simulink library "SimWindFarm_lib"  (Simulink 10.3)
settings: Solver=ode45  StartTime=0.0  StopTime=10.0  RelTol=1e-3  EnableMultiTasking=on
undefined symbols (not defined in the file): sigbuilder_block
libraries: simulink x3
(part 2 of 2)

== system SimWindFarm_lib/Farm Template - No Taylor Added Turbulence/Post processing ==
  Fatigue Computation : Subsystem
      settings: OpenFcn=fatigue=fatiguegui(logsout);
      mask Display: image(imread('rainflow.png'))

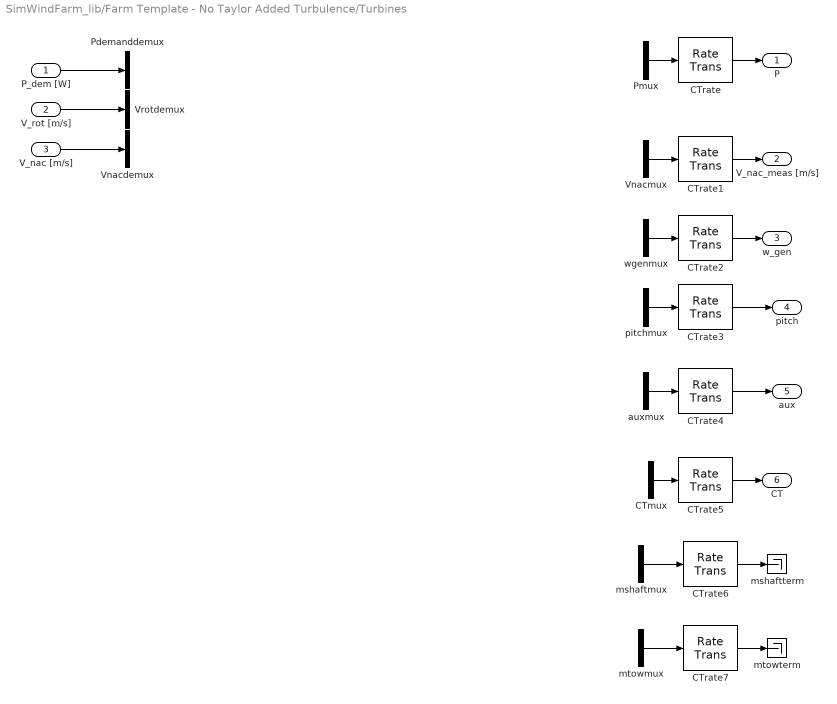
== system SimWindFarm_lib/Farm Template - No Taylor Added Turbulence/Turbines ==
  P_dem [W] : Inport
  V_rot [m/s] : Inport  Port=2
  V_nac [m/s] : Inport  Port=3
  CTmux : Mux  Inputs=2
  CTrate{,1..7} (8 alike) : RateTransition  Deterministic=off  OutPortSampleTime=TTs
  Pdemanddemux : Demux  Outputs=3
  Pmux : Mux  Inputs=2
  Vnacdemux : Demux  Outputs=3
  Vnacmux : Mux  Inputs=2
  Vrotdemux : Demux  Outputs=3
  auxmux : Mux  Inputs=2
  mshaftmux : Mux  Inputs=2
  mshaftterm : Terminator
  mtowmux : Mux  Inputs=2
  mtowterm : Terminator
  pitchmux : Mux  Inputs=2
  wgenmux : Mux  Inputs=2
  P : Outport
  V_nac_meas [m/s] : Outport  Port=2
  w_gen : Outport  Port=3
  pitch : Outport  Port=4
  aux : Outport  Port=5
  CT : Outport  Port=6
  wires:
  V_nac [m/s]/1 -> Vnacdemux/1
  P_dem [W]/1 -> Pdemanddemux/1
  V_rot [m/s]/1 -> Vrotdemux/1
  Pmux/1 -> CTrate/1
  CTmux/1 -> CTrate5/1
  Vnacmux/1 -> CTrate1/1
  pitchmux/1 -> CTrate3/1
  auxmux/1 -> CTrate4/1
  wgenmux/1 -> CTrate2/1
  mshaftmux/1 -> CTrate6/1
  mtowmux/1 -> CTrate7/1
  CTrate/1 -> P/1
  CTrate1/1 -> V_nac_meas [m/s]/1
  CTrate2/1 -> w_gen/1
  CTrate3/1 -> pitch/1
  CTrate4/1 -> aux/1
  CTrate5/1 -> CT/1
  CTrate6/1 -> mshaftterm/1
  CTrate7/1 -> mtowterm/1

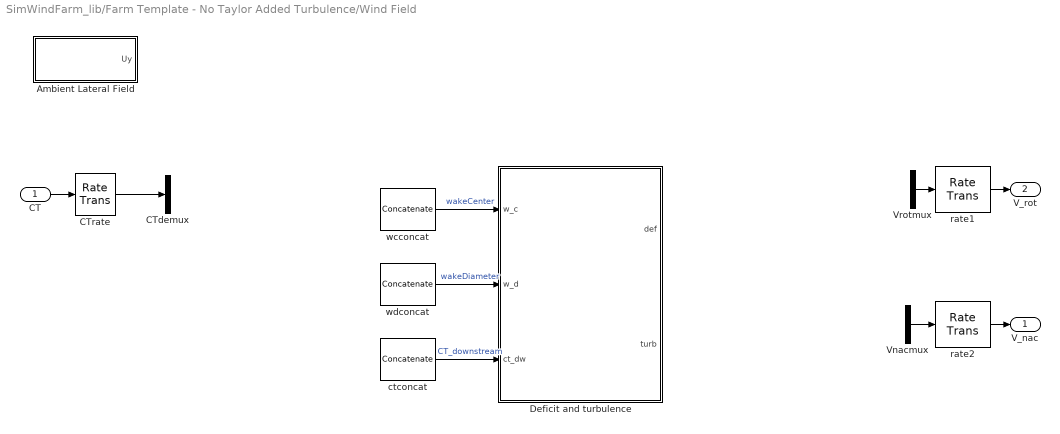
== system SimWindFarm_lib/Farm Template - No Taylor Added Turbulence/Wind Field ==
  CT : Inport
  Ambient Lateral Field : Subsystem
      mask init:
      | wind=get_param(gcb,'UserData');
  CTdemux : Demux  Outputs=3
  CTrate : RateTransition  Deterministic=off  OutPortSampleTime=10
  Deficit and turbulence : MATLAB Function  TreatAsAtomicUnit=on
  Vnacmux : Mux  Inputs=2
  Vrotmux : Mux  Inputs=2
  ctconcat : Concatenate  Mode=Multidimensional array  ConcatenateDimension=2
  rate1 : RateTransition  Deterministic=off  OutPortSampleTime=SWFTTs
  rate2 : RateTransition  Deterministic=off  OutPortSampleTime=SWFTTs
  wcconcat : Concatenate  Mode=Multidimensional array  ConcatenateDimension=2
  wdconcat : Concatenate  Mode=Multidimensional array  ConcatenateDimension=2
  V_nac : Outport
  V_rot : Outport  Port=2
  wires:
  rate2/1 -> V_nac/1
  rate1/1 -> V_rot/1
  Vnacmux/1 -> rate2/1
  Vrotmux/1 -> rate1/1
  ctconcat/1 -> Deficit and turbulence/3(ct_dw)  "CT_downstream"
  wdconcat/1 -> Deficit and turbulence/2(w_d)  "wakeDiameter"
  wcconcat/1 -> Deficit and turbulence/1(w_c)  "wakeCenter"
  CT/1 -> CTrate/1
  CTrate/1 -> CTdemux/1

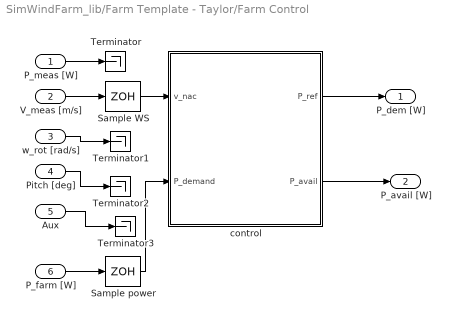
== system SimWindFarm_lib/Farm Template - Taylor/Farm Control ==
  P_meas [W] : Inport
  V_meas [m/s] : Inport  Port=2
  w_rot [rad/s] : Inport  Port=3
  Pitch [deg] : Inport  Port=4
  " Aux" : Inport  Port=5
  P_farm [W] : Inport  Port=6
  Sample WS : ZeroOrderHold  SampleTime=CTs
  Sample power : ZeroOrderHold  SampleTime=CTs
  Terminator{,1..3} (4 alike) : Terminator
  control : MATLAB Function  TreatAsAtomicUnit=on
  P_dem [W] : Outport
  P_avail [W] : Outport  Port=2
  wires:
  P_farm [W]/1 -> Sample power/1
  control/1(P_ref) -> P_dem [W]/1
  control/2(P_avail) -> P_avail [W]/1
  Sample power/1 -> control/2(P_demand)
  V_meas [m/s]/1 -> Sample WS/1
  Sample WS/1 -> control/1(v_nac)
  P_meas [W]/1 -> Terminator/1
  w_rot [rad/s]/1 -> Terminator1/1
  Pitch [deg]/1 -> Terminator2/1
  " Aux"/1 -> Terminator3/1

== system SimWindFarm_lib/Farm Template - Taylor/Grid ==
  Generated Power [W] : Inport
  Consumed Power [W] : Inport  Port=2
  Active power diff to freq : Gain  Gain=frequencygain
  Integrator : Integrator  InitialCondition=50  LimitOutput=on  UpperSaturationLimit=100  LowerSaturationLimit=0
  Sum1 : Sum  Inputs=|+-
  Grid Frequency [Hz] : Outport
  wires:
  Integrator/1 -> Grid Frequency [Hz]/1
  Sum1/1 -> Active power diff to freq/1
  Active power diff to freq/1 -> Integrator/1
  Generated Power [W]/1 -> Sum1/1
  Consumed Power [W]/1 -> Sum1/2

== system SimWindFarm_lib/Farm Template - Taylor/Network Load ==
  Power Load : Subsystem  Tag=STV Subsys  LoadFcn=sigbuilder_block('load');  StartFcn=sigbuilder_block('start');  StopFcn=sigbuilder_block('stop');  ClipboardFcn=sigbuilder_block('clipboard');  mask(Sigbuilder block){tuvar=[0:10]}
      mask help: Sigbuilder GUI
      mask init:
      | if ~strcmp(get_param(bdroot(gcbh),'SimulationStatus'),'stopped') tuvar = sigbuilder_block('maskInit'); end
      settings: CopyFcn=sigbuilder_block('copy');  DeleteFcn=sigbuilder_block('delete');  ModelCloseFcn=sigbuilder_block('modelClose');  PreSaveFcn=sigbuilder_block('preSave');  PauseFcn=sigbuilder_block('pause')  ContinueFcn=sigbuilder_block('continue')  NameChangeFcn=sigbuilder_block('namechange');  OpenFcn=sigbuilder_block('open',[437.6 199.2 550.4 400 ]);  CloseFcn=sigbuilder_block('close');
      mask Display: plot(0, 0, 100, 100,[2, 2, 32, 32, 2], [68, 8, 8, 68, 68],[32, 2], [38, 38], [32, 19, 2],[53, 60, 44], [32, 17, 17, 2],[16, 16, 31, 31]);txt = getActiveGroup(gcbh);text(2, 100, txt,'verticalAlignment', 'top');
  To rated farm power : Gain  Gain=maxpower
  Power Consumption [W] : Outport
  wires:
  Power Load/1(Signal 1) -> To rated farm power/1
  To rated farm power/1 -> Power Consumption [W]/1

== system SimWindFarm_lib/Farm Template - Taylor/Network Operator ==
  P_avail [W] : Inport
  Freq [Hz] : Inport  Port=2
  F_meas delay : TransportDelay  DelayTime=parm.delay
  Network Operator : MATLAB Function  TreatAsAtomicUnit=on
  P meas delay : TransportDelay  DelayTime=parm.delay
  Reference delay : TransportDelay  DelayTime=.01
  Sample frequency : ZeroOrderHold  SampleTime=parm.Ts
  Sample power : ZeroOrderHold  SampleTime=parm.Ts
  Unit Delay : UnitDelay  SampleTime=parm.Ts  HasFrameUpgradeWarning=on
  settings : Constant  Value=parm.settings  OutDataTypeStr=double  SampleTime=parm.Ts
  P_farm [W] : Outport
  wires:
  Freq [Hz]/1 -> Sample frequency/1
  Unit Delay/1 -> Network Operator/4(P_demand0)
  Sample frequency/1 -> F_meas delay/1  "f"
  settings/1 -> Network Operator/2(settings)  "settings"
  Sample power/1 -> P meas delay/1
  P_avail [W]/1 -> Sample power/1
  Network Operator/1(P_demand) -> Unit Delay/1, Reference delay/1
  F_meas delay/1 -> Network Operator/3(f)
  P meas delay/1 -> Network Operator/1(P_avail)
  Reference delay/1 -> P_farm [W]/1

== system SimWindFarm_lib/Farm Template - Taylor/Post processing ==
  Fatigue Computation : Subsystem
      settings: OpenFcn=fatigue=fatiguegui(logsout);
      mask Display: image(imread('rainflow.png'))
  Wake Animation : Subsystem
      settings: OpenFcn=|
      | sys=bdroot(gcb);
      | create_wakeanim(sys,logsout);
      mask Display: image(imread('wakeanim.png'))
  Wind Field Animation : Subsystem
      settings: OpenFcn=|
      | sys=bdroot(gcb);
      | windanim(sys,logsout);
      mask Display: image(imread('windanim.png'))

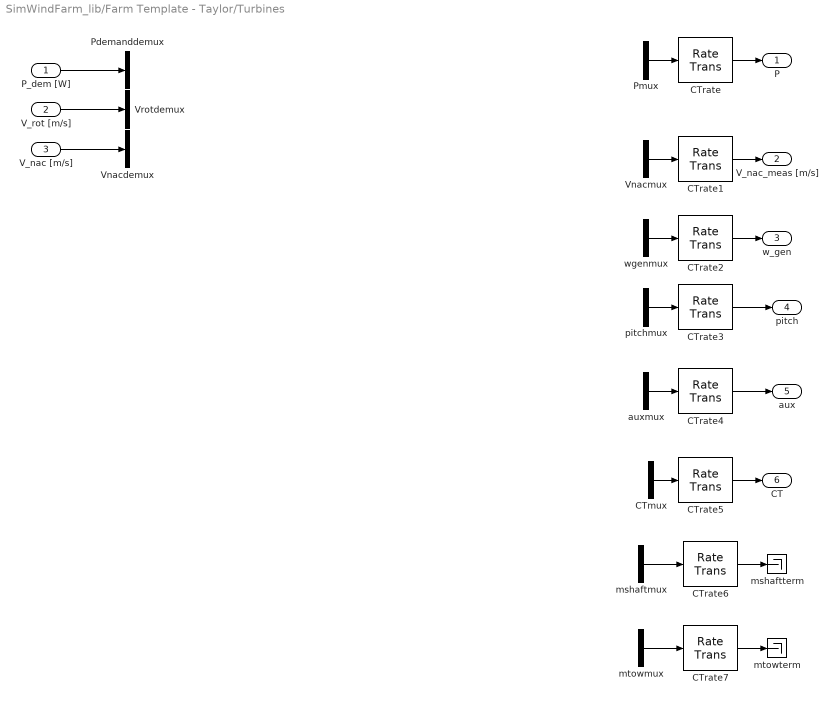
== system SimWindFarm_lib/Farm Template - Taylor/Turbines ==
  P_dem [W] : Inport
  V_rot [m/s] : Inport  Port=2
  V_nac [m/s] : Inport  Port=3
  CTmux : Mux  Inputs=2
  CTrate{,1..7} (8 alike) : RateTransition  Deterministic=off  OutPortSampleTime=TTs
  Pdemanddemux : Demux  Outputs=3
  Pmux : Mux  Inputs=2
  Vnacdemux : Demux  Outputs=3
  Vnacmux : Mux  Inputs=2
  Vrotdemux : Demux  Outputs=3
  auxmux : Mux  Inputs=2
  mshaftmux : Mux  Inputs=2
  mshaftterm : Terminator
  mtowmux : Mux  Inputs=2
  mtowterm : Terminator
  pitchmux : Mux  Inputs=2
  wgenmux : Mux  Inputs=2
  P : Outport
  V_nac_meas [m/s] : Outport  Port=2
  w_gen : Outport  Port=3
  pitch : Outport  Port=4
  aux : Outport  Port=5
  CT : Outport  Port=6
  wires:
  V_nac [m/s]/1 -> Vnacdemux/1
  P_dem [W]/1 -> Pdemanddemux/1
  V_rot [m/s]/1 -> Vrotdemux/1
  Pmux/1 -> CTrate/1
  CTmux/1 -> CTrate5/1
  Vnacmux/1 -> CTrate1/1
  pitchmux/1 -> CTrate3/1
  auxmux/1 -> CTrate4/1
  wgenmux/1 -> CTrate2/1
  mshaftmux/1 -> CTrate6/1
  mtowmux/1 -> CTrate7/1
  CTrate/1 -> P/1
  CTrate1/1 -> V_nac_meas [m/s]/1
  CTrate2/1 -> w_gen/1
  CTrate3/1 -> pitch/1
  CTrate4/1 -> aux/1
  CTrate5/1 -> CT/1
  CTrate6/1 -> mshaftterm/1
  CTrate7/1 -> mtowterm/1

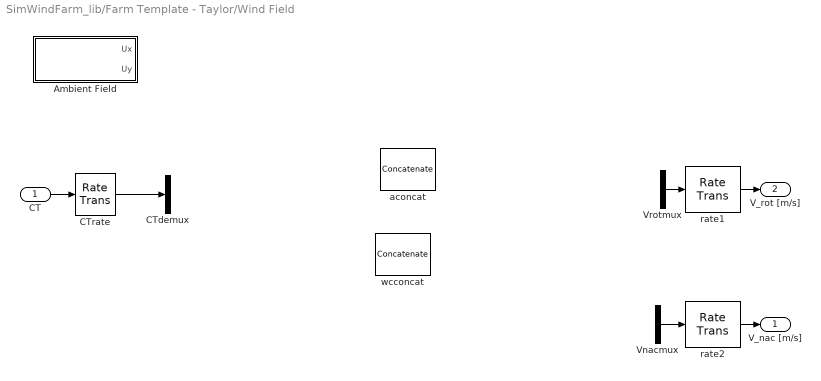
== system SimWindFarm_lib/Farm Template - Taylor/Wind Field ==
  CT : Inport
  Ambient Field : Subsystem
      mask init:
      | wind=get_param(gcb,'UserData');
  CTdemux : Demux  Outputs=3
  CTrate : RateTransition  Deterministic=off  OutPortSampleTime=10
  Vnacmux : Mux  Inputs=2
  Vrotmux : Mux  Inputs=2
  aconcat : Concatenate  Mode=Multidimensional array  ConcatenateDimension=2
  rate1 : RateTransition  Deterministic=off  OutPortSampleTime=SWFTTs
  rate2 : RateTransition  Deterministic=off  OutPortSampleTime=SWFTTs
  wcconcat : Concatenate  Mode=Multidimensional array  ConcatenateDimension=2
  V_nac [m/s] : Outport
  V_rot [m/s] : Outport  Port=2
  wires:
  CT/1 -> CTrate/1
  Vrotmux/1 -> rate1/1
  Vnacmux/1 -> rate2/1
  CTrate/1 -> CTdemux/1
  rate1/1 -> V_rot [m/s]/1
  rate2/1 -> V_nac [m/s]/1

== system SimWindFarm_lib/Farm Template - No Taylor/Network Load/Power Load ==
  Demux : Demux  Tag=STV Demux  Outputs=1
      settings: DisplayOption=none
  FromWs : FromWorkspace  Tag=STV FromWs  VariableName=tuvar  SigBuilderData=DataTag0  VnvData=DataTag1
      SigBuilderData=|
      | common.afterFinalStr = 'Extrapolate'
      | common.sampleTime = 0
      | dataSet.timeRange = [0 1000]
      | dataSet.name = 'Group 1'
      | sbobj.Groups.Name = 'Group 1'
      | sbobj.Groups.Signals.Name = 'Signal 1'
      | sbobj.Groups.Signals.XData = [0 25 100 200 500 1000]
      | sbobj.Groups.Signals.YData = [0.1 0.1 0.7 0.7 0.9 0.85]
  Signal 1 : Outport  Tag=STV Outport
  wires:
  FromWs/1 -> Demux/1
  Demux/1 -> Signal 1/1

== system SimWindFarm_lib/Farm Template - No Taylor/Post processing/Fatigue Computation ==

== system SimWindFarm_lib/Farm Template - No Taylor/Wind Field/Ambient Lateral Field ==
  Counter Free-Running : simulink/Sources/Counter Free-Running  NumBits=32  tsamp=wind.Ts
  Selector1 : Selector  NumberOfDimensions=2  InputPortWidth=3  IndexOptions=Select all,Index vector (port)  Indices=[1 3],1  OutputSizes=1,1
  Sum : Sum  Inputs=|++
  Turb x : Constant  Value=ceil(wind.grid.xsize/wind.grid.size)-wind.xgrids
  Uy_full : Constant  Value=wind.Uy
  Uy : Outport
  wires:
  Uy_full/1 -> Selector1/1
  Sum/1 -> Selector1/2
  Counter Free-Running/1 -> Sum/2
  Turb x/1 -> Sum/1
  Selector1/1 -> Uy/1

== system SimWindFarm_lib/Farm Template - No Taylor Added Turbulence/Network Load/Power Load ==
  Demux : Demux  Tag=STV Demux  Outputs=1
      settings: DisplayOption=none
  FromWs : FromWorkspace  Tag=STV FromWs  VariableName=tuvar  SigBuilderData=DataTag2  VnvData=DataTag3
      SigBuilderData=|
      | common.afterFinalStr = 'Extrapolate'
      | common.sampleTime = 0
      | dataSet.timeRange = [0 1000]
      | dataSet.name = 'Group 1'
      | sbobj.Groups.Name = 'Group 1'
      | sbobj.Groups.Signals.Name = 'Signal 1'
      | sbobj.Groups.Signals.XData = [0 25 100 200 500 1000]
      | sbobj.Groups.Signals.YData = [0.1 0.1 0.7 0.7 0.9 0.85]
  Signal 1 : Outport  Tag=STV Outport
  wires:
  Demux/1 -> Signal 1/1
  FromWs/1 -> Demux/1

== system SimWindFarm_lib/Farm Template - No Taylor Added Turbulence/Post processing/Fatigue Computation ==

== system SimWindFarm_lib/Farm Template - No Taylor Added Turbulence/Wind Field/Ambient Lateral Field ==
  Counter Free-Running : simulink/Sources/Counter Free-Running  NumBits=32  tsamp=wind.Ts
  Selector1 : Selector  NumberOfDimensions=2  InputPortWidth=3  IndexOptions=Select all,Index vector (port)  Indices=[1 3],1  OutputSizes=1,1
  Sum : Sum  Inputs=|++
  Turb x : Constant  Value=ceil(wind.grid.xsize/wind.grid.size)-wind.xgrids
  Uy_full : Constant  Value=wind.Uy
  Uy : Outport
  wires:
  Selector1/1 -> Uy/1
  Turb x/1 -> Sum/1
  Counter Free-Running/1 -> Sum/2
  Sum/1 -> Selector1/2
  Uy_full/1 -> Selector1/1

== system SimWindFarm_lib/Farm Template - Taylor/Network Load/Power Load ==
  Demux : Demux  Tag=STV Demux  Outputs=1
      settings: DisplayOption=none
  FromWs : FromWorkspace  Tag=STV FromWs  VariableName=tuvar  SigBuilderData=DataTag4  VnvData=DataTag5
      SigBuilderData=|
      | common.afterFinalStr = 'Extrapolate'
      | common.sampleTime = 0
      | dataSet.timeRange = [0 1000]
      | dataSet.name = 'Group 1'
      | sbobj.Groups.Name = 'Group 1'
      | sbobj.Groups.Signals.Name = 'Signal 1'
      | sbobj.Groups.Signals.XData = [0 25 100 200 500 1000]
      | sbobj.Groups.Signals.YData = [0.1 0.1 0.7 0.7 0.9 0.85]
  Signal 1 : Outport  Tag=STV Outport
  wires:
  Demux/1 -> Signal 1/1
  FromWs/1 -> Demux/1

== system SimWindFarm_lib/Farm Template - Taylor/Post processing/Fatigue Computation ==

== system SimWindFarm_lib/Farm Template - Taylor/Post processing/Wake Animation ==

== system SimWindFarm_lib/Farm Template - Taylor/Post processing/Wind Field Animation ==

== system SimWindFarm_lib/Farm Template - Taylor/Wind Field/Ambient Field ==
  Counter Free-Running : simulink/Sources/Counter Free-Running  NumBits=32  tsamp=wind.Ts
  Selector : Selector  NumberOfDimensions=2  InputPortWidth=3  IndexOptions=Select all,Index vector (port)  Indices=[1 3],1  OutputSizes=1,1
  Selector1 : Selector  NumberOfDimensions=2  InputPortWidth=3  IndexOptions=Select all,Index vector (port)  Indices=[1 3],1  OutputSizes=1,1
  Sum : Sum  Inputs=|++
  Turb x : Constant  Value=ceil(wind.grid.xsize/wind.grid.size)-wind.xgrids
  Ux_full : Constant  Value=wind.Ux
  Uy_full : Constant  Value=wind.Uy
  Ux : Outport
  Uy : Outport  Port=2
  wires:
  Selector/1 -> Ux/1
  Selector1/1 -> Uy/1
  Turb x/1 -> Sum/1
  Counter Free-Running/1 -> Sum/2
  Sum/1 -> Selector/2, Selector1/2
  Uy_full/1 -> Selector1/1
  Ux_full/1 -> Selector/1

== matlab function Farm Template - No Taylor/Farm Control/control ==
  data: v_nac input double; P_demand input double; parm parameter double; P_ref output double; P_avail output double
function [P_ref,P_avail]  = Farm_Controller(v_nac,P_demand,parm)
%
% Farm_Controller estimates the available power at the farm and distributes the 
% power references proportional to the available power at each wind turbine.
%
% [P_ref,P_avail_total]  = Farm_Controller(v_nac,P_demand)
%
% vn : the wind speed at wind turbine number n.
%
% P_demand : The demanded power by the operator.
%
% P_ref : The power reference for the wind turbines.
%
% P_avail : Available power at the farm level
%
%
% Version 1: 2009-04-10 sms
% Version 2: 2009-12-04 grunnet
% By : S. Mohsen N. Soltani & Jacob D. Grunnet
% Aalborg University, Dept. of Electronic Systems, Section of Automation
% and Control
% E-mail: sms@es.aau.dk
% E-mail: grunnet@es.aau.dk

rho=parm.rho; %air dencity
R=parm.radius; %rotor radius
rated=parm.rated; %Rated power
N=parm.N; %Number of turbines
Cp=parm.Cp; % Max cp of the turbines

P_a=zeros(N,1);
P_ref=zeros(N,1);

% Compute available power at each turbine
for i=1:N
    %P_a=1/2*pi*r^2*Cp*v^3
    P_a(i)=min(rated(i),(pi/2)*rho*R(i)^2*v_nac(i)^3*Cp(i));
end

%Compute total available power
P_avail=sum(P_a);

%Distribute power according to availibility
for i=1:N
    P_ref(i)=max(0,min(rated(i),P_demand*P_a(i)/P_avail));
end

== matlab function Farm Template - No Taylor/Network Operator/Network Operator ==
  data: P_avail input double; settings input double; f input double; P_demand output double; P_demand0 input double; parm parameter double
function P_demand = TSO(P_avail,settings,f,P_demand0,parm)
%
% TSO provides the demanded power to the wind farm controller.
%
% P_avail : Aavailable power at the farm level.
%
% mode : The operation mode.
%
% settings : The settings corresponding to the operational mode
%
% f : Frequency of the network
%
% P_deamnd0 : The last update of the deamded power
%
% Ts : Sample Time
%
% Time-stamp: <2009-04-10 sms>
% Version 1: 2009-04-10 sms 
% By : S. Mohsen N. Soltani
% Aalborg University, Dept. of Electronic Systems, Section of Automation
% and Control
% E-mail: sms@es.aau.dk
% 
 P=0;
 switch(parm.mode)
     case 1 %Absolute active power control
        P=settings(1);
%       % type='Full power';
     case 2 %Delta mode
        P=P_avail-settings(1);
%       % type='Delta mode';
     case 3 %Balance
        P=settings(1);
%       % type='Balance';
     case 4 %Rate limiter
        P=min(P_avail,settings(1)*parm.Ts+P_demand0);
%       % type='Rate limiter';
     case 5 %Frequency Control
        deadb=settings(1);
        contb=settings(2);
        maxp=settings(3);
        minp=settings(4);
        f=f-settings(5); % To provide Delta f
        if ( f<= deadb && f>=-deadb)
            P=0.5*(maxp+minp);
        elseif f>= contb
            P=minp;
        elseif f<= -contb
            P=maxp;
        elseif ( f>deadb && f<contb)
            P=0.5*(maxp+minp)-0.5*(maxp-minp)*(f-deadb)/(contb-deadb);
        elseif ( f<-deadb && f>-contb)
            P=0.5*(maxp+minp)-0.5*(maxp-minp)*(f+deadb)/(contb-deadb);
        end
%       % type='Frequency Control';
     otherwise %Unknown
        P=P_avail;
%       % type='Unknown Mode';
 end
%        

P_demand=max(0,P);

== matlab function Farm Template - No Taylor/Wind Field/Deficit ==
  data: w_c input double; w_d input double; ct_dw input double; p parameter double; def output double; turb output double
function [def, turb] = deficit(w_c,w_d,ct_dw,p) %#eml
% w_c   is the vector of wake centers from the other turbins at the x position of the turbine
% w_d   is the vector of wake diameters from the other turbins at the x position of the turbine
% ct_dw is the vector of thrust coefficients from the other turbins at the x position of the turbine
% p     is a structure containing farm layout and tubine rotor sizes  

wake_from = zeros(length(p.farm.x),length(p.farm.x));
dist_i = zeros(length(p.farm.x),1);
def = ones(length(p.farm.x),1);
turb = ones(length(p.farm.x),1);

if ct_dw(size(ct_dw,1),1) ~= 0 % only calculate deficit if wind has reached end of farm
    [~, dist_i] = sort(p.farm.x);

    %This for-loop make a "tree" of which turbines are in the wake
    for i=1:length(p.farm.x)
        turb_i = dist_i(i);
        for k = 1:length(p.farm.x)
            turb_k = dist_i(k);
            temp = p.farm.y(turb_k)-w_c(turb_k,turb_i);
            %if turb_k is in turb_i's wake it is included in the "tree"
            if(temp > -w_d(turb_k,turb_i) && temp < w_d(turb_k,turb_i))  
                wake_from(i,k) = 1; %
            end
        end
    end
    wake_from_2 = wake_from; %copy original wake tree for later use

    for i=1:length(p.farm.x)
        % remove parents from tree if children is in wake = use iterative scheme
        pp = find(wake_from(:,i)==1);
        c = find(wake_from(i,:)==1);
        wake_from(pp,c) = 0;
        switch length(pp)
            case 0 % if no wake the deficit is one    %similar for 'turbulence gain'
                def(i) = 1;
                turb(i) = 1;
            case 1 % if one wake then calculate deficit using iterative scheme
                wake_upstream = find(wake_from_2(:,i)==1); %find the upstream turbines
                wd = w_d(dist_i(i),dist_i(min(wake_upstream))); %find wake diameter for "most" upstream turbine
                tmp_ct = ct_dw(dist_i(i),dist_i(max(wake_upstream))); % find CT for closest upstream turbine
                tmp_rotor_D = 2*p.rotor.r(dist_i(max(wake_upstream))); % precalculate rotor diameter for closest upstream turbine
                if(length(wake_upstream) == 1) % if only one upstream turbine use "normal" deficit calculation
                    def(i) = 1-0.5*tmp_rotor_D^2/wd^2*tmp_ct;
                else % else use iterative scheme : "Analytical Modelling of Wind Speed Deficit in Large Offshore Wind Farms" eq:17
                    tmp_def = def(max(wake_upstream)); %find deficit at closest upstream turbine
                    tmp_D = w_d(dist_i(max(wake_upstream)),dist_i(min(wake_upstream))); %find diameter of wake at closest upstream turbine
                    def(i) = 1-(tmp_D^2/wd^2*(1-tmp_def)+0.5*tmp_rotor_D^2/wd^2*tmp_ct*tmp_def); %calculate deficit
                end
            otherwise % if more than wakes meet (overlap but not in row) merge according to area
                %error = 1 % uncomment to see when wakes are merged from other rows
                wake_upstream = find(wake_from_2(:,i)==1);
                wd = w_d(dist_i(i),dist_i(min(wake_upstream)));
                tmp_def = ones(length(pp),1);
                tmp_D = ones(length(pp),1);
                k = 1;
                for l=length(pp) %calculate deficit from each upstream turbine
                    j = pp(l);
                    tmp_ct = ct_dw(dist_i(i),dist_i(j));
                    tmp_def_up = def(dist_i(j));
                    tmp_rotor_D = 2*p.rotor.r(dist_i(max(wake_upstream)));
                    tmp_D(k) = w_d(dist_i(j),dist_i(min(wake_upstream)));
                    tmp_def(k) = 1-(tmp_D(k)^2/wd^2*(1-tmp_def_up)+0.5*tmp_rotor_D^2/wd^2*tmp_ct*tmp_def_up);
                    k = k+1;
                end
                def(i) = sum(tmp_D.^2.*tmp_def)/sum(tmp_D.^2); %combine deficit according to area
        end
    end
    def(dist_i) = def; % Reshuffle deficits such that turbine number is correct
end

== matlab function Farm Template - No Taylor Added Turbulence/Farm Control/control ==
  data: v_nac input double; P_demand input double; parm parameter double; P_ref output double; P_avail output double
function [P_ref,P_avail]  = Farm_Controller(v_nac,P_demand,parm)
%
% Farm_Controller estimates the available power at the farm and distributes the 
% power references proportional to the available power at each wind turbine.
%
% [P_ref,P_avail_total]  = Farm_Controller(v_nac,P_demand)
%
% vn : the wind speed at wind turbine number n.
%
% P_demand : The demanded power by the operator.
%
% P_ref : The power reference for the wind turbines.
%
% P_avail : Available power at the farm level
%
%
% Version 1: 2009-04-10 sms
% Version 2: 2009-12-04 grunnet
% By : S. Mohsen N. Soltani & Jacob D. Grunnet
% Aalborg University, Dept. of Electronic Systems, Section of Automation
% and Control
% E-mail: sms@es.aau.dk
% E-mail: grunnet@es.aau.dk

rho=parm.rho; %air dencity
R=parm.radius; %rotor radius
rated=parm.rated; %Rated power
N=parm.N; %Number of turbines
Cp=parm.Cp; % Max cp of the turbines

P_a=zeros(N,1);
P_ref=zeros(N,1);

% Compute available power at each turbine
for i=1:N
    %P_a=1/2*pi*r^2*Cp*v^3
    P_a(i)=min(rated(i),(pi/2)*rho*R(i)^2*v_nac(i)^3*Cp(i));
end

%Compute total available power
P_avail=sum(P_a);

%Distribute power according to availibility
for i=1:N
    P_ref(i)=max(0,min(rated(i),P_demand*P_a(i)/P_avail));
end

== matlab function Farm Template - No Taylor Added Turbulence/Network Operator/Network Operator ==
  data: P_avail input double; settings input double; f input double; P_demand output double; P_demand0 input double; parm parameter double
function P_demand = TSO(P_avail,settings,f,P_demand0,parm)
%
% TSO provides the demanded power to the wind farm controller.
%
% P_avail : Aavailable power at the farm level.
%
% mode : The operation mode.
%
% settings : The settings corresponding to the operational mode
%
% f : Frequency of the network
%
% P_deamnd0 : The last update of the deamded power
%
% Ts : Sample Time
%
% Time-stamp: <2009-04-10 sms>
% Version 1: 2009-04-10 sms 
% By : S. Mohsen N. Soltani
% Aalborg University, Dept. of Electronic Systems, Section of Automation
% and Control
% E-mail: sms@es.aau.dk
% 
 P=0;
 switch(parm.mode)
     case 1 %Absolute active power control
        P=settings(1);
%       % type='Full power';
     case 2 %Delta mode
        P=P_avail-settings(1);
%       % type='Delta mode';
     case 3 %Balance
        P=settings(1);
%       % type='Balance';
     case 4 %Rate limiter
        P=min(P_avail,settings(1)*parm.Ts+P_demand0);
%       % type='Rate limiter';
     case 5 %Frequency Control
        deadb=settings(1);
        contb=settings(2);
        maxp=settings(3);
        minp=settings(4);
        f=f-settings(5); % To provide Delta f
        if ( f<= deadb && f>=-deadb)
            P=0.5*(maxp+minp);
        elseif f>= contb
            P=minp;
        elseif f<= -contb
            P=maxp;
        elseif ( f>deadb && f<contb)
            P=0.5*(maxp+minp)-0.5*(maxp-minp)*(f-deadb)/(contb-deadb);
        elseif ( f<-deadb && f>-contb)
            P=0.5*(maxp+minp)-0.5*(maxp-minp)*(f+deadb)/(contb-deadb);
        end
%       % type='Frequency Control';
     otherwise %Unknown
        P=P_avail;
%       % type='Unknown Mode';
 end
%        

P_demand=max(0,P);

== matlab function Farm Template - No Taylor Added Turbulence/Wind Field/Deficit and turbulence ==
  data: w_c input double; w_d input double; ct_dw input double; p parameter double; def output double; turb output double
function [def, turb] = deficit(w_c,w_d,ct_dw,p) %#eml
% w_c   is the vector of wake centers from the other turbins at the x position of the turbine
% w_d   is the vector of wake diameters from the other turbins at the x position of the turbine
% ct_dw is the vector of thrust coefficients from the other turbins at the x position of the turbine
% p     is a structure containing farm layout and tubine rotor sizes  

wake_from = zeros(length(p.farm.x),length(p.farm.x));
dist_i = zeros(length(p.farm.x),1);
def = ones(length(p.farm.x),1);

turb = ones(length(p.farm.x),1);
sigma0 = p.sigma0; %ambient wind speed turbulence intensity
U0 = p.U0; %ambient wind speed mean 

if ct_dw(size(ct_dw,1),1) ~= 0 % only calculate deficit if wind has reached end of farm
    [~, dist_i] = sort(p.farm.x);

    %This for-loop make a "tree" of which turbines are in the wake
    for i=1:length(p.farm.x)
        turb_i = dist_i(i);
        for k = 1:length(p.farm.x)
            turb_k = dist_i(k);
            temp = p.farm.y(turb_k)-w_c(turb_k,turb_i);
            %if turb_k is in turb_i's wake it is included in the "tree"
            if(temp > -w_d(turb_k,turb_i) && temp < w_d(turb_k,turb_i))  
                wake_from(i,k) = 1; %
            end
        end
    end
    wake_from_2 = wake_from; %copy original wake tree for later use

    for i=1:length(p.farm.x)
        % remove parents from tree if children is in wake = use iterative scheme
        pp = find(wake_from(:,i)==1);
        c = find(wake_from(i,:)==1);
        wake_from(pp,c) = 0;
        switch length(pp)
            case 0 % if no wake the deficit/turbulence is one
                def(i) = 1;
                turb(i) = 1;
            case 1 % if one wake then calculate deficit using iterative scheme
                wake_upstream = find(wake_from_2(:,i)==1); %find the upstream turbines
                wd = w_d(dist_i(i),dist_i(min(wake_upstream))); %find wake diameter for "most" upstream turbine
                tmp_ct = ct_dw(dist_i(i),dist_i(max(wake_upstream))); % find CT for closest upstream turbine
                tmp_rotor_D = 2*p.rotor.r(dist_i(max(wake_upstream))); % precalculate rotor diameter for closest upstream turbine
                if(length(wake_upstream) == 1) % if only one upstream turbine use "normal" deficit calculation
                    def(i) = 1-0.5*tmp_rotor_D^2/wd^2*tmp_ct;
                else % else use iterative scheme : "Analytical Modelling of Wind Speed Deficit in Large Offshore Wind Farms" eq:17
                    tmp_def = def(max(wake_upstream)); %find deficit at closest upstream turbine
                    tmp_D = w_d(dist_i(max(wake_upstream)),dist_i(min(wake_upstream))); %find diameter of wake at closest upstream turbine
                    def(i) = 1-(tmp_D^2/wd^2*(1-tmp_def)+0.5*tmp_rotor_D^2/wd^2*tmp_ct*tmp_def); %calculate deficit
                end
                    
                %Euclidean distance Edist between turbine in wake and closest wake generating turbine
                Edist = sqrt((p.farm.x(dist_i(i)) - p.farm.x(dist_i(max(wake_upstream))))^2 + ...
                (p.farm.y(dist_i(i)) - p.farm.y(dist_i(max(wake_upstream))))^2);
                %added turbulence sigma_add, eq (4.14) in Frandsen thesis
                sigma_add = (U0*def(i))/(1.5 + 0.8*((Edist/tmp_rotor_D)/sqrt(abs(tmp_ct)))); 
                %added turbulence scaling parameter turb, rearranged from
                %eq (3.17) in Frandsen such that sigma_Turbine = turb*sigma0
                turb(i) = sqrt((sigma_add/(sigma0*U0))^2 + 1); %we multiply with U0 in denominator since sigma0 is actually ambient turbulence intensity
            otherwise % if more than wakes meet (overlap but not in row) merge according to area
                %error = 1 % uncomment to see when wakes are merged from other rows
                wake_upstream = find(wake_from_2(:,i)==1);
                wd = w_d(dist_i(i),dist_i(min(wake_upstream)));
                tmp_def = ones(length(pp),1);
                tmp_D = ones(length(pp),1);
                
                tmp_turb = ones(length(pp),1);
                k = 1;
                for l=length(pp) %calculate deficit from each upstream turbine
                    j = pp(l);
                    tmp_ct = ct_dw(dist_i(i),dist_i(j));
                    tmp_def_up = def(dist_i(j));
                    tmp_rotor_D = 2*p.rotor.r(dist_i(max(wake_upstream)));
                    tmp_D(k) = w_d(dist_i(j),dist_i(min(wake_upstream)));
                    tmp_def(k) = 1-(tmp_D(k)^2/wd^2*(1-tmp_def_up)+0.5*tmp_rotor_D^2/wd^2*tmp_ct*tmp_def_up);
 
                    k = k+1;
                end
                def(i) = sum(tmp_D.^2.*tmp_def)/sum(tmp_D.^2); %combine deficit according to area
                k = 1;
                for l=length(pp) %calculate deficit from each upstream turbine
                    j = pp(l);
                    tmp_ct = ct_dw(dist_i(i),dist_i(j));
                    
                    Edist = sqrt((p.farm.x(dist_i(i)) - p.farm.x(dist_i(j)))^2 + ...
                    (p.farm.y(dist_i(i)) - p.farm.y(dist_i(j)))^2);%should dist_i(j) be dist_i(max(wake_upstream)) here?
                    tmp_rotor_D_turb = 2*p.rotor.r(dist_i(j));
                    sigma_add = (U0*def(i))/(1.5 + 0.8*((Edist/tmp_rotor_D_turb)/sqrt(abs(tmp_ct))));
                    tmp_turb(k) = sqrt((sigma_add/(sigma0*U0))^2 + 1); %we multiply with U0 in denominator since sigma0 is actually ambient turbulence intensity
                    k = k+1;
                end
                turb(i) = sum(tmp_D.^2.*tmp_turb)/sum(tmp_D.^2); %combine turbulence according to area
        end
    end
    def(dist_i) = def; % Reshuffle deficits/turbulence such that turbine number is correct
    turb(dist_i) = turb;
end

== matlab function Farm Template - Taylor/Farm Control/control ==
  data: v_nac input double; P_demand input double; parm parameter double; P_ref output double; P_avail output double
function [P_ref,P_avail]  = Farm_Controller(v_nac,P_demand,parm)
%
% Farm_Controller estimates the available power at the farm and distributes the 
% power references proportional to the available power at each wind turbine.
%
% [P_ref,P_avail_total]  = Farm_Controller(v_nac,P_demand)
%
% vn : the wind speed at wind turbine number n.
%
% P_demand : The demanded power by the operator.
%
% P_ref : The power reference for the wind turbines.
%
% P_avail : Available power at the farm level
%
%
% Version 1: 2009-04-10 sms
% Version 2: 2009-12-04 grunnet
% By : S. Mohsen N. Soltani & Jacob D. Grunnet
% Aalborg University, Dept. of Electronic Systems, Section of Automation
% and Control
% E-mail: sms@es.aau.dk
% E-mail: grunnet@es.aau.dk

rho=parm.rho; %air dencity
R=parm.radius; %rotor radius
rated=parm.rated; %Rated power
N=parm.N; %Number of turbines
Cp=parm.Cp; % Max cp of the turbines

P_a=zeros(N,1);
P_ref=zeros(N,1);

% Compute available power at each turbine
for i=1:N
    %P_a=1/2*pi*r^2*Cp*v^3
    P_a(i)=min(rated(i),(pi/2)*rho*R(i)^2*v_nac(i)^3*Cp(i));
end

%Compute total available power
P_avail=sum(P_a);

%Distribute power according to availibility
for i=1:N
    P_ref(i)=max(0,min(rated(i),P_demand*P_a(i)/P_avail));
end

== matlab function Farm Template - Taylor/Network Operator/Network Operator ==
  data: P_avail input double; settings input double; f input double; P_demand output double; P_demand0 input double; parm parameter double
function P_demand = TSO(P_avail,settings,f,P_demand0,parm)
%
% TSO provides the demanded power to the wind farm controller.
%
% P_avail : Aavailable power at the farm level.
%
% mode : The operation mode.
%
% settings : The settings corresponding to the operational mode
%
% f : Frequency of the network
%
% P_deamnd0 : The last update of the deamded power
%
% Ts : Sample Time
%
% Time-stamp: <2009-04-10 sms>
% Version 1: 2009-04-10 sms 
% By : S. Mohsen N. Soltani
% Aalborg University, Dept. of Electronic Systems, Section of Automation
% and Control
% E-mail: sms@es.aau.dk
% 
 P=0;
 switch(parm.mode)
     case 1 %Absolute active power control
        P=settings(1);
%       % type='Full power';
     case 2 %Delta mode
        P=P_avail-settings(1);
%       % type='Delta mode';
     case 3 %Balance
        P=settings(1);
%       % type='Balance';
     case 4 %Rate limiter
        P=min(P_avail,settings(1)*parm.Ts+P_demand0);
%       % type='Rate limiter';
     case 5 %Frequency Control
        deadb=settings(1);
        contb=settings(2);
        maxp=settings(3);
        minp=settings(4);
        f=f-settings(5); % To provide Delta f
        if ( f<= deadb && f>=-deadb)
            P=0.5*(maxp+minp);
        elseif f>= contb
            P=minp;
        elseif f<= -contb
            P=maxp;
        elseif ( f>deadb && f<contb)
            P=0.5*(maxp+minp)-0.5*(maxp-minp)*(f-deadb)/(contb-deadb);
        elseif ( f<-deadb && f>-contb)
            P=0.5*(maxp+minp)-0.5*(maxp-minp)*(f+deadb)/(contb-deadb);
        end
%       % type='Frequency Control';
     otherwise %Unknown
        P=P_avail;
%       % type='Unknown Mode';
 end
%        

P_demand=max(0,P);
